simulink model "PWMSynthesizer"  (R2020a)
settings: Solver=VariableStepAuto  StartTime=0.0  StopTime=1  RelTol=1e-3
libraries: ee_lib x6, fl_lib x3, nesl_utility x2, dspvision x1
settings Model: Creator=yukikamatani  LastModifiedBy=yukikamatani

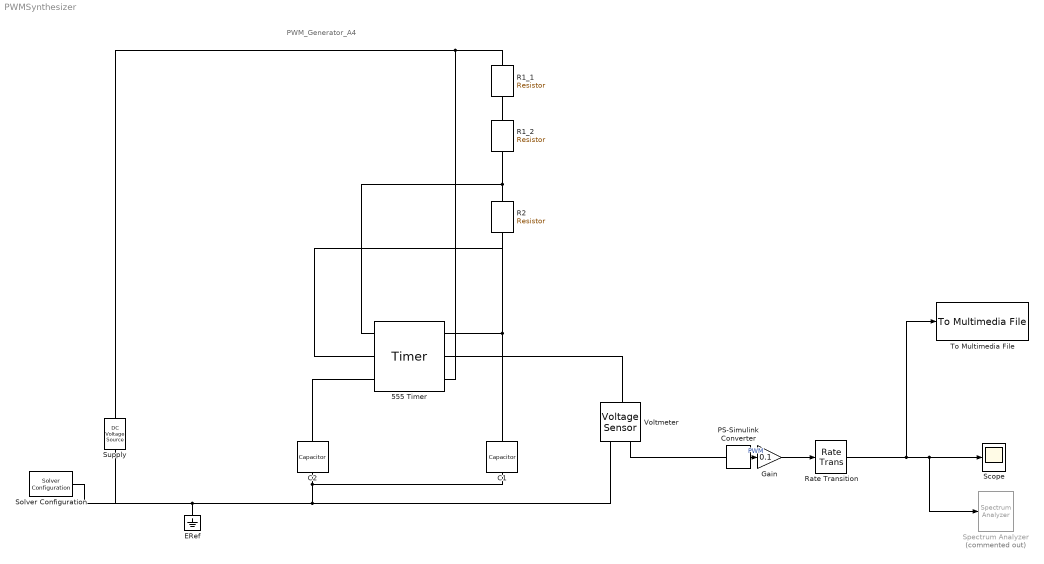
== system PWMSynthesizer ==
  note: PWM_Generator_A4
  555 Timer : ee_lib/Integrated Circuits/Timer  V_CC=5 V  V_OL=0 V  V_OH=5 V  R_OUT=8 Ohm  Delay=1e-7 s  R_DIV=5 kOhm  R_closed=12 Ohm  R_open=5e+8 Ohm
      settings: AttributesFormatString=Vcc = %<V_CC>V  SourceProductBaseCode=PS  InternalSimscapePortConfiguration="{\"Bottom\":[],\"Left\":[{\"id\":\"TRIG\",\"label\":\"TRIG\",\"type\":\"foundation.electrical.electrical\"},{\"id\":\"OUT\",\"label\":\"OUT\",\"type\":\"foundation.electrical.electrical\"},{\"id\":\"RESET\",\"label\":\"RESET\",\"type\":\"foundation.electrical.electrical\"}],\"Right\":[{\"id\":\"DISCH\",\"label\":\"DISCH\",\"type\":\"foundation.electrical.electrical\"},{\"id\":\"THRES\",\"label\":\"THRES\",\"type\":\"foundation.electrical.electrical\"},{\"id\":\"CONT\",\"label\":\"CONT\",\"type\":\"foundation.electrical.electrical\"}],\"Top\":[]}"
  C1 : ee_lib/Passive/Capacitor  cap_option=0  c=0.1 uF  Cvec=[ 1e-5 1e-6 ] F  Vvec=[ 0 10 ] V  CV_table_symmetry=1  f_vec=[1, 10] kHz  DFext_vec=[.8, 1.2]  C_tol=5  enable_C_tol=0  tol_distribution=1  nSigma=4  r=1e-6 Ohm  g=0 1/Ohm  averaging_period=0 s  enable_operating_limits=0  operating_limit_action=2  max_working_voltage_range=[ -25 25 ] V  power_rating=1 W  enable_faults=0  fault_action=1  Cscale_faulted=100  R_faulted=0.001 Ohm  G_faulted=0 1/Ohm  tau_fault=0.001 s  enable_temporal_fault=0  t_fault=1 s  enable_behavioral_fault=0  max_permissible_voltage_range=[ -100 100 ] V  t_fail_on_voltage=1 s  i_specify=off  i_priority=None  i=0 A  i_nominal_specify=off  i_nominal_unit=A  i_nominal_value=1  v_specify=off  v_priority=None  v=0 V  v_nominal_specify=off  v_nominal_unit=V  v_nominal_value=1  vc_specify=on  vc_priority=High  vc=0 V  vc_nominal_specify=off  vc_nominal_unit=V  vc_nominal_value=1
      settings: AttributesFormatString=%<c>%<c_unit>
  C2 : ee_lib/Passive/Capacitor  cap_option=0  c=10 nF  Cvec=[ 1e-5 1e-6 ] F  Vvec=[ 0 10 ] V  CV_table_symmetry=1  f_vec=[1, 10] kHz  DFext_vec=[.8, 1.2]  C_tol=5  enable_C_tol=0  tol_distribution=1  nSigma=4  r=1e-6 Ohm  g=0 1/Ohm  averaging_period=0 s  enable_operating_limits=0  operating_limit_action=2  max_working_voltage_range=[ -25 25 ] V  power_rating=1 W  enable_faults=0  fault_action=1  Cscale_faulted=100  R_faulted=0.001 Ohm  G_faulted=0 1/Ohm  tau_fault=0.001 s  enable_temporal_fault=0  t_fault=1 s  enable_behavioral_fault=0  max_permissible_voltage_range=[ -100 100 ] V  t_fail_on_voltage=1 s  i_specify=off  i_priority=None  i=0 A  i_nominal_specify=off  i_nominal_unit=A  i_nominal_value=1  v_specify=off  v_priority=None  v=0 V  v_nominal_specify=off  v_nominal_unit=V  v_nominal_value=1  vc_specify=on  vc_priority=High  vc=0 V  vc_nominal_specify=off  vc_nominal_unit=V  vc_nominal_value=1
      settings: AttributesFormatString=%<c>%<c_unit>
  ERef : fl_lib/Electrical/Electrical Elements/Electrical Reference
      settings: SourceProductBaseCode=MT,SS
  Gain : Gain  Gain=0.1
  PS-Simulink Converter : nesl_utility/PS-Simulink Converter  PhysicalDomain=network_engine_domain  SubClassName=ps_output  LeftPortType=input  RightPortType=output  PseudoPeriodic=off  Frequencies=[]  Unit=1  AffineConversion=off
      settings: SourceProductBaseCode=MT,SS
  R1_1 : ee_lib/Passive/Resistor  R=2.7 kOhm  R_tol=5  enable_R_tol=0  tol_distribution=1  nSigma=4  enable_operating_limits=0  operating_limit_action=2  max_working_voltage=100 V  power_rating=1 W  enable_faults=0  fault_action=1  R_faulted=Inf Ohm  enable_temporal_fault=0  t_fault=1 s  enable_behavioral_fault=0  max_permissible_current=1 A  t_fail_on_current=1 s  noise_mode=0  sample_time=0.001 s  repeatability=1  auto_seed=3243031446  user_seed=0  Tdevice=25 degC  alpha=3.93e-3 1/K  Tmeas=25 degC  thermal_mass=100 J/K  power_derating_T1=70 degC  power_derating_T2=155 degC  operating_temperature_range_vec=[-50, 150] degC  temperature_specify=off  temperature_priority=High  temperature=298.15 K  temperature_nominal_specify=off  temperature_nominal_unit=K  temperature_nominal_value=1
      settings: AttributesFormatString=%<R>%<R_unit>
  R1_2 : ee_lib/Passive/Resistor  R=560 Ohm  R_tol=5  enable_R_tol=0  tol_distribution=1  nSigma=4  enable_operating_limits=0  operating_limit_action=2  max_working_voltage=100 V  power_rating=1 W  enable_faults=0  fault_action=1  R_faulted=Inf Ohm  enable_temporal_fault=0  t_fault=1 s  enable_behavioral_fault=0  max_permissible_current=1 A  t_fail_on_current=1 s  noise_mode=0  sample_time=0.001 s  repeatability=1  auto_seed=3256068099  user_seed=0  Tdevice=25 degC  alpha=3.93e-3 1/K  Tmeas=25 degC  thermal_mass=100 J/K  power_derating_T1=70 degC  power_derating_T2=155 degC  operating_temperature_range_vec=[-50, 150] degC  temperature_specify=off  temperature_priority=High  temperature=298.15 K  temperature_nominal_specify=off  temperature_nominal_unit=K  temperature_nominal_value=1
      settings: AttributesFormatString=%<R>%<R_unit>
  R2 : ee_lib/Passive/Resistor  R=15 kOhm  R_tol=5  enable_R_tol=0  tol_distribution=1  nSigma=4  enable_operating_limits=0  operating_limit_action=2  max_working_voltage=100 V  power_rating=1 W  enable_faults=0  fault_action=1  R_faulted=Inf Ohm  enable_temporal_fault=0  t_fault=1 s  enable_behavioral_fault=0  max_permissible_current=1 A  t_fail_on_current=1 s  noise_mode=0  sample_time=0.001 s  repeatability=1  auto_seed=1620901523  user_seed=0  Tdevice=25 degC  alpha=3.93e-3 1/K  Tmeas=25 degC  thermal_mass=100 J/K  power_derating_T1=70 degC  power_derating_T2=155 degC  operating_temperature_range_vec=[-50, 150] degC  temperature_specify=off  temperature_priority=High  temperature=298.15 K  temperature_nominal_specify=off  temperature_nominal_unit=K  temperature_nominal_value=1
      settings: AttributesFormatString=%<R>%<R_unit>
  Rate Transition : RateTransition  OutPortSampleTime=1/44100
      settings: AttributesFormatString=SampleTime = %<OutPortSampleTime>[sec]
  Scope : Scope
  Solver Configuration : nesl_utility/Solver Configuration  PhysicalDomain=network_engine_domain  SubClassName=solver  LeftPortType=input  RightPortType=generic  Tones=[]  Harmonics=[]  SimulateNoise=off  Profile=off  UseLocalSampling=off  EnableSwitchedLinearOptims=on  FrequencyDomain=off  UseCCode=off  RelTol=0.001  AbsTol=1e-06  MinStep=1e-09  ToWorkspace=off  RevertToSquareIcSolve=off  NumHomotopyIterations=100  PhasorMode=off  PhasorModeNumHarmonics=1  DoDC=off  ResidualTolerance=1e-10  UseLocalSolver=off  LocalSolverChoice=NE_BACKWARD_EULER_ADVANCER  LocalSolverSampleTime=0.001  DoFixedCost=off  MaxNonlinIter=3  MaxModeIter=2  LinearAlgebra=auto  EquationFormulation=NE_TIME_EF  DelaysMemoryBudget=1024  AutomaticFiltering=on  FilteringTimeConstant=0.001  PartitionStorageMethod=AS_NEEDED  PartitionMemoryBudget=1024  PartitionMethod=FAST
      settings: SourceProductBaseCode=MT,SS
  Spectrum Analyzer : SpectrumAnalyzer  Commented=on
  Supply : fl_lib/Electrical/Electrical Sources/DC Voltage Source  v0=5 V
      settings: AttributesFormatString=%<v0>V  SourceProductBaseCode=MT,SS
  To Multimedia File : dspvision/To Multimedia File  outputFilename=output.wav  streamSelection=Audio only  videoCompressor=None (uncompressed)  audioCompressor=None (uncompressed)  imagePorts=Separate color signals  fileType=WAV  audioDatatype=16-bit integer  fourcc=RGB  videoQuality=75  mj2000CompFactor=10
  Voltmeter : fl_lib/Electrical/Electrical Sensors/Voltage Sensor
      settings: SourceProductBaseCode=MT,SS
  wires:
  Rate Transition/1 -> Scope/1, Spectrum Analyzer/1, To Multimedia File/1
  Gain/1 -> Rate Transition/1
  PS-Simulink Converter/1 -> Gain/1  "PWM"
  connections:
  C2/RConn1 -- Voltmeter/RConn2 -- Supply/RConn1 -- Solver Configuration/RConn1 -- ERef/LConn1 -- C1/RConn1
  PS-Simulink Converter/LConn1 -- Voltmeter/RConn1
  R1_1/RConn1 -- Supply/LConn1 -- 555 Timer/LConn3
  555 Timer/LConn2 -- Voltmeter/LConn1
  R1_2/RConn1 -- R1_1/LConn1
  555 Timer/LConn1 -- 555 Timer/RConn2 -- R2/LConn1 -- C1/LConn1
  C2/LConn1 -- 555 Timer/RConn3
  R2/RConn1 -- 555 Timer/RConn1 -- R1_2/LConn1
